simulink model "lab_2"  (R2021b)
settings: Solver=ode4  StartTime=0.0  StopTime=60  FixedStep=0.001  RelTol=1e-3
settings Model: Creator=egorkashirov  LastModifiedBy=andrey
settings SolverCC: AlgebraicLoopSolver=TrustRegion
settings DebuggingCC: SFMachineParentedDataDiag=warning

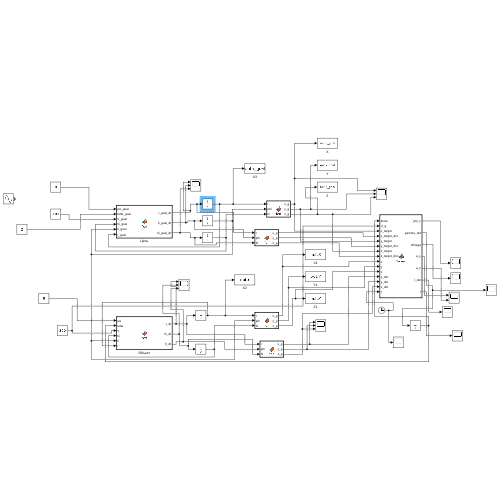
[thumbnail: Simulink's stored preview of the top-level diagram]
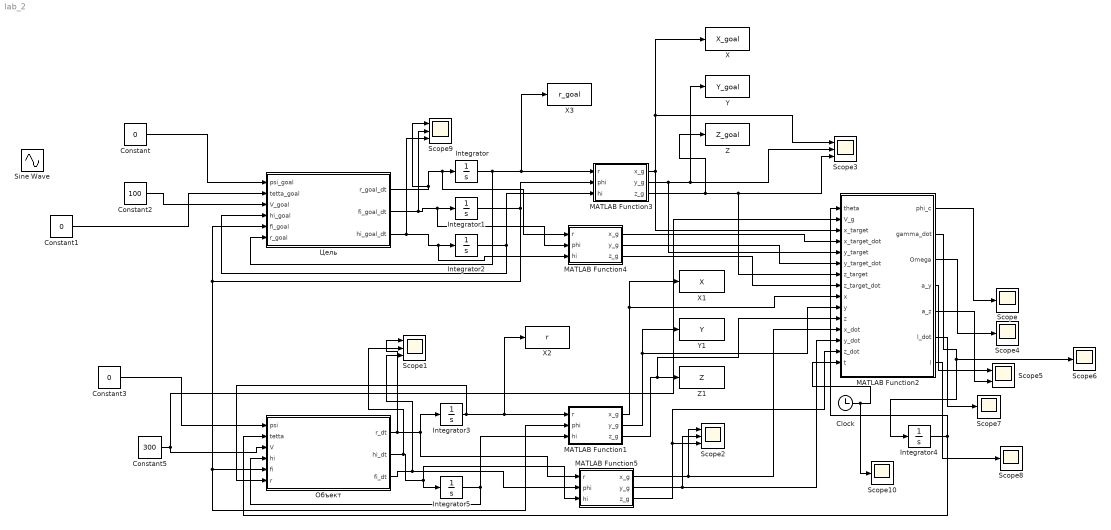
== system lab_2 ==
  Clock : Clock
  Constant : Constant  Value=0
  Constant1 : Constant  Value=0
  Constant2 : Constant  Value=100
  Constant3 : Constant  Value=0
  Constant5 : Constant  Value=300
  Integrator : Integrator  InitialCondition=2000
  Integrator1 : Integrator  InitialCondition=pi/4
  Integrator2 : Integrator  InitialCondition=0.001
  Integrator3 : Integrator  InitialCondition=1
  Integrator4 : Integrator  InitialCondition=pi/6
  Integrator5 : Integrator  InitialCondition=0.001
  MATLAB Function1 : MATLAB Function  TreatAsAtomicUnit=on
  MATLAB Function2 : MATLAB Function  TreatAsAtomicUnit=on
  MATLAB Function3 : MATLAB Function  TreatAsAtomicUnit=on
  MATLAB Function4 : MATLAB Function  TreatAsAtomicUnit=on
  MATLAB Function5 : MATLAB Function  TreatAsAtomicUnit=on
  Scope{,4,6..8,10} (6 alike) : Scope
  Scope{1..3,9} (4 alike) : Scope  NumInputPorts=3
  Scope5 : Scope  NumInputPorts=2
  Sine Wave : Sin  Amplitude=0.8  Frequency=0.5  Phase=pi/2  SampleTime=0
  X : ToWorkspace  VariableName=X_goal  SaveFormat=Timeseries  SampleTime=-1
  X1 : ToWorkspace  VariableName=X  SaveFormat=Timeseries  SampleTime=-1
  X2 : ToWorkspace  VariableName=r  SaveFormat=Timeseries  SampleTime=-1
  X3 : ToWorkspace  VariableName=r_goal  SaveFormat=Timeseries  SampleTime=-1
  Y : ToWorkspace  VariableName=Y_goal  SaveFormat=Timeseries  SampleTime=-1
  Y1 : ToWorkspace  VariableName=Y  SaveFormat=Timeseries  SampleTime=-1
  Z : ToWorkspace  VariableName=Z_goal  SaveFormat=Timeseries  SampleTime=-1
  Z1 : ToWorkspace  VariableName=Z  SaveFormat=Timeseries  SampleTime=-1
  Объект : MATLAB Function  TreatAsAtomicUnit=on
  Цель : MATLAB Function  TreatAsAtomicUnit=on
  wires:
  Constant/1 -> Цель/1(psi_goal)
  Constant2/1 -> Цель/3(V_goal)
  Цель/1(r_goal_dt) -> Scope9/1, MATLAB Function4/1(r), Integrator/1
  Цель/2(fi_goal_dt) -> Scope9/2, MATLAB Function4/2(phi), Integrator1/1
  Цель/3(hi_goal_dt) -> MATLAB Function4/3(hi), Integrator2/1, Scope9/3
  Integrator2/1 -> MATLAB Function3/3(hi), Цель/4(hi_goal)
  Integrator1/1 -> Цель/5(fi_goal), Объект/5(fi), MATLAB Function1/2(phi), MATLAB Function3/2(phi)
  Integrator/1 -> Цель/6(r_goal), X3/1, MATLAB Function3/1(r)
  MATLAB Function3/1(x_g) -> X/1, Scope3/1, MATLAB Function2/3(x_target)
  MATLAB Function3/2(y_g) -> Scope3/2, Y/1, MATLAB Function2/5(y_target)
  MATLAB Function3/3(z_g) -> MATLAB Function2/7(z_target), Scope3/3, Z/1
  Constant5/1 -> Объект/3(V), MATLAB Function2/2(V_g)
  Объект/2(hi_dt) -> Scope1/2, Integrator5/1, MATLAB Function5/3(hi)
  Integrator3/1 -> Объект/6(r), X2/1, MATLAB Function1/1(r)
  Integrator5/1 -> MATLAB Function1/3(hi), Объект/4(hi)
  Объект/1(r_dt) -> Scope1/1, Integrator3/1, MATLAB Function5/1(r)
  MATLAB Function1/1(x_g) -> X1/1, MATLAB Function2/9(x)
  MATLAB Function1/2(y_g) -> MATLAB Function2/10(y), Y1/1
  Constant3/1 -> Объект/1(psi)
  MATLAB Function1/3(z_g) -> MATLAB Function2/11(z), Z1/1
  Constant1/1 -> Цель/2(tetta_goal)
  MATLAB Function4/1(x_g) -> MATLAB Function2/4(x_target_dot)
  MATLAB Function4/2(y_g) -> MATLAB Function2/6(y_target_dot)
  MATLAB Function4/3(z_g) -> MATLAB Function2/8(z_target_dot)
  Объект/3(fi_dt) -> Scope1/3, MATLAB Function5/2(phi)
  MATLAB Function5/1(x_g) -> Scope2/1, MATLAB Function2/12(x_dot)
  MATLAB Function5/2(y_g) -> Scope2/2, MATLAB Function2/13(y_dot)
  MATLAB Function5/3(z_g) -> Scope2/3, MATLAB Function2/14(z_dot)
  MATLAB Function2/2(gamma_dot) -> Scope6/1, Integrator4/1
  Integrator4/1 -> Объект/2(tetta), MATLAB Function2/1(theta)
  MATLAB Function2/1(phi_c) -> Scope/1
  MATLAB Function2/3(Omega) -> Scope4/1
  MATLAB Function2/4(a_y) -> Scope5/1
  MATLAB Function2/5(a_z) -> Scope5/2
  MATLAB Function2/6(l_dot) -> Scope7/1
  MATLAB Function2/7(l) -> Scope8/1
  Clock/1 -> Scope10/1, MATLAB Function2/15(t)

== matlab function lab_2/MATLAB Function4 ==
  data: r input; x_g output; phi input; hi input; y_g output; z_g output
function [x_g, y_g, z_g] = fcn(r, phi, hi)
    x_g = r* cos(phi)*cos(hi);
    y_g = r*sin(phi);
    z_g = -r*cos(phi)*sin(hi);
end

== matlab function lab_2/MATLAB Function5 ==
  data: r input; x_g output; phi input; hi input; y_g output; z_g output
function [x_g, y_g, z_g] = fcn(r, phi, hi)
    x_g = r* cos(phi)*cos(hi);
    y_g = r*sin(phi);
    z_g = -r*cos(phi)*sin(hi);
end

== matlab function lab_2/MATLAB Function1 ==
  data: r input; x_g output; phi input; hi input; y_g output; z_g output
function [x_g, y_g, z_g] = fcn(r, phi, hi)
    x_g = r* cos(phi)*cos(hi);
    y_g = r*sin(phi);
    z_g = -r*cos(phi)*sin(hi);
end

== matlab function lab_2/Цель ==
  data: psi_goal input; r_goal_dt output; tetta_goal input; V_goal input; hi_goal input; fi_goal input; fi_goal_dt output; hi_goal_dt output; r_goal input
function [r_goal_dt, fi_goal_dt, hi_goal_dt] = fcn(psi_goal,tetta_goal,V_goal,hi_goal,fi_goal,r_goal)

r_goal_dt = V_goal*cos(tetta_goal)*cos(psi_goal-hi_goal)*cos(fi_goal)+V_goal*sin(tetta_goal)*sin(fi_goal);
fi_goal_dt = (-V_goal*cos(tetta_goal)*cos(psi_goal-hi_goal)*sin(fi_goal)+V_goal*sin(tetta_goal)*cos(fi_goal))/r_goal;
hi_goal_dt = (V_goal*cos(tetta_goal)*sin(psi_goal-hi_goal))/r_goal/cos(fi_goal);

end

== matlab function lab_2/Объект ==
  data: psi input; r_dt output; tetta input; V input; hi input; fi input; hi_dt output; r input; fi_dt output
function [r_dt, hi_dt, fi_dt] = fcn(psi,tetta,V,hi,fi,r)

r_dt = V*cos(tetta)*cos(psi-hi)*cos(fi)+V*sin(tetta)*sin(fi);
fi_dt = (-V*cos(tetta)*cos(psi-hi)*sin(fi)+V*sin(tetta)*cos(fi))/r;
%hi_dt = (V*cos(tetta)*sin(psi-hi))/r/cos(fi);
hi_dt = (V*cos(tetta)*sin(psi-hi))/r/cos(fi);

end

== matlab function lab_2/MATLAB Function3 ==
  data: r input; x_g output; phi input; hi input; y_g output; z_g output
function [x_g, y_g, z_g] = fcn(r, phi, hi)
    x_g = r* cos(phi)*cos(hi);
    y_g = r*sin(phi);
    z_g = -r*cos(phi)*sin(hi);
end

== matlab function lab_2/MATLAB Function2 ==
  data: theta input; phi_c output; V_g input; x_target input; x_target_dot input; y_target input; y_target_dot input; z_target input; z_target_dot input; x input; y input; z input; x_dot input; y_dot input; z_dot input; gamma_dot output; Omega output; a_y output; a_z output; l_dot output; l output; t input
function [phi_c, gamma_dot, Omega, a_y, a_z, l_dot, l] = Naved(theta, V_g, x_target, x_target_dot, y_target, y_target_dot, z_target, z_target_dot, x, y, z, x_dot, y_dot, z_dot, t)
    delay = 2;
    if t < delay
        gamma_dot = 0;
        phi_c = 0; Omega = [0 0 0]'; a_y = 0; a_z = 0; l_dot = [0 0 0]'; l = [0 0 0]';
    else
    
        mu = 1;
        N = 100;
    
        l = [x_target y_target z_target]' - [x y z]';
        l_dot = [x_target_dot y_target_dot z_target_dot]' - [x_dot y_dot z_dot]';
        l_n = norm(l);
%         l_dot_n = norm(l_dot);
        R_g_v2 = [cos(theta) sin(theta) 0; -sin(theta) cos(theta) 0; 0 0 1];
        Omega = R_g_v2 * cross(l/l_n, l_dot/l_n);
    %Omega = cross(l/l_n, l_dot/l_n);
    
        a_y = mu*N*V_g*Omega(3);
        a_z = -mu*N*V_g*Omega(2);
    
    %     phi_c = atan(a_z/abs(a_y));
        phi_c = 1;
        gamma_dot = sign(a_y)/V_g*sqrt(a_y^2+a_z^2);
       % gamma_dot = sign(a_z)/V_g*sqrt(a_y^2+a_z^2);
    %    k = 1;
    %    gamma_dot = k * Omega(3) * V_g;
    %    gamma_dot = 0.001;
    end

end
